simulink model "tanquenolineal"  (R2021a)
settings: Solver=VariableStepAuto  StartTime=0.0  StopTime=10.0  RelTol=1e-3
settings Model: Creator=guille  LastModifiedBy=guille

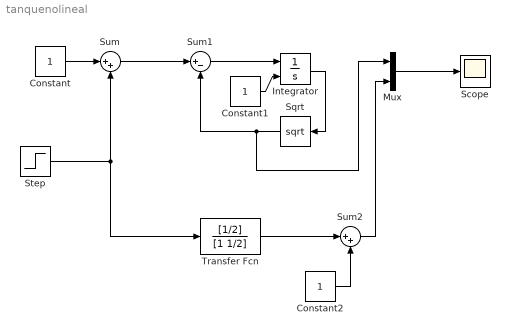
== system tanquenolineal ==
  Constant : Constant
  Constant1 : Constant
  Constant2 : Constant
  Integrator : Integrator  InitialConditionSource=external
  Mux : Mux  Inputs=2
  Scope : Scope
  Sqrt : Sqrt  SaturateOnIntegerOverflow=on
  Step : Step  After=0.1  SampleTime=0
  Sum : Sum  Inputs=|++
  Sum1 : Sum  Inputs=|+-
  Sum2 : Sum  Inputs=|++
  Transfer Fcn : TransferFcn  Numerator=[1/2]  Denominator=[1 1/2]
  wires:
  Mux/1 -> Scope/1
  Integrator/1 -> Sqrt/1
  Sum1/1 -> Integrator/1
  Constant1/1 -> Integrator/2
  Sqrt/1 -> Sum1/2, Mux/1
  Constant/1 -> Sum/1
  Step/1 -> Transfer Fcn/1, Sum/2
  Sum/1 -> Sum1/1
  Transfer Fcn/1 -> Sum2/1
  Sum2/1 -> Mux/2
  Constant2/1 -> Sum2/2
